simulink model "gm_sampleModel1406_3_sub"  (R2023a)
settings: Solver=VariableStepAuto  StartTime=0.0  StopTime=10.0  RelTol=1e-3
libraries: hdlsllib x2
settings Model: Creator=user1  LastModifiedBy=user1
settings OptimizationCC: BlockReduction=off  ConditionallyExecuteInputs=off
settings DebuggingCC: InheritedTsInSrcMsg=none

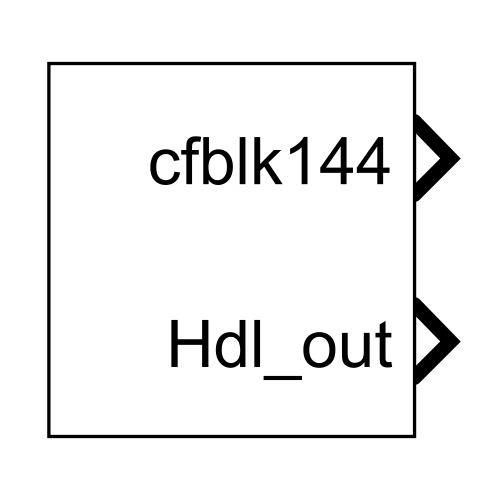
[thumbnail: Simulink's stored preview of the top-level diagram]
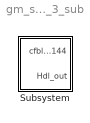
== system gm_sampleModel1406_3_sub ==
  Subsystem : Subsystem

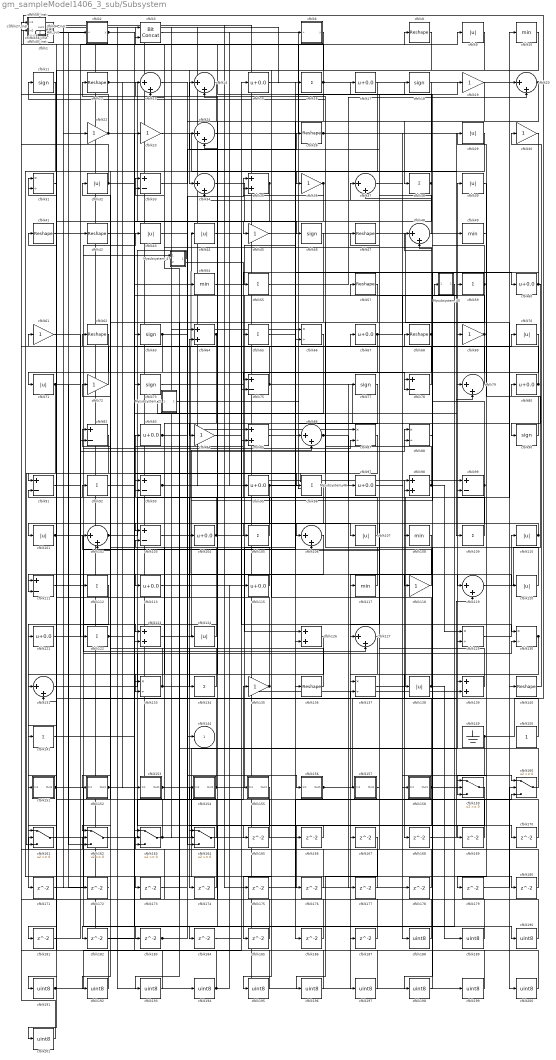
== system gm_sampleModel1406_3_sub/Subsystem ==
  Mysubsystem_21 : Subsystem
  Mysubsystem_40 : Subsystem
  Mysubsystem_46 : Subsystem
  Mysubsystem_47 : Subsystem
  cfblk1 : hdlsllib/Logic and Bit Operations/Interval Test  IntervalClosedRight=on  uplimit=0.5  IntervalClosedLeft=on  lowlimit=-0.5  OutDataTypeStr=uint8
  cfblk{10,49,54,108,117} (5 alike) : MinMax  OutDataTypeStr=uint8
  cfblk{9,29,32,39,43..44,70..71,101,107,110,120,124,138} (14 alike) : Abs  OutDataTypeStr=uint8  SaturateOnIntegerOverflow=off
  cfblk{13..14,20,24,34,37,48,79,86,102,106,119,127,131} (14 alike) : Sum  Inputs=|++  OutDataTypeStr=uint8
  cfblk{33,75,78,82,91,93,99,103,111} (9 alike) : Sum  Inputs=+-  OutDataTypeStr=uint8
  cfblk{15,17,60,67,80,83,95,97,104,113,115,121} (12 alike) : Bias  Bias=0.0  SaturateOnIntegerOverflow=off
  cfblk{16,38,55,59,65,92,96,105,109,112,122,134,141} (13 alike) : Sum  Inputs=+  OutDataTypeStr=uint8
  cfblk{11,18,46,63,73,77,90} (7 alike) : Signum
  cfblk114_inst : Subsystem
  cfblk116_inst : Subsystem
  cfblk{19,22..23,30,36,45,61,69,72,84,118,135} (12 alike) : Gain  OutDataTypeStr=uint8
  cfblk{8,12,26,41..42,47,57,62,68,136,140} (11 alike) : Reshape
  cfblk{35,64,85,98,123,126,139} (7 alike) : Sum  OutDataTypeStr=uint8
  cfblk128_inst : Subsystem
  cfblk{31,66,87..88,129..130,133,137} (8 alike) : Product  Inputs=*/  OutDataTypeStr=uint8  RndMeth=Zero  SaturateOnIntegerOverflow=on
  cfblk132_inst : Subsystem
  cfblk149 : Ground
  cfblk150 : Constant  OutDataTypeStr=uint8  SampleTime=-1
  cfblk151 : Subsystem
  cfblk152 : Subsystem
  cfblk153 : Subsystem
  cfblk154 : Subsystem
  cfblk155 : Subsystem
  cfblk156 : Subsystem
  cfblk157 : Subsystem
  cfblk158 : Subsystem
  cfblk{159..164} (6 alike) : Switch  OutDataTypeStr=uint8  SaturateOnIntegerOverflow=off  InputSameDT=off
  cfblk{165..187} (23 alike) : Delay  SampleTime=1
  cfblk{188..201} (14 alike) : DataTypeConversion  OutDataTypeStr=uint8  SaturateOnIntegerOverflow=off  RndMeth=Floor
  cfblk2 : Subsystem  mask(Compare To Constant){relop=<=, const=double(3), OutDataTypeStr=uint8, ZeroCross=on}
      mask prompts: relop "Simulink:masks:Operator_MP"; const "Simulink:masks:ConstantValue_MP"; OutDataTypeStr "Simulink:masks:OutputDataType_MP"; ZeroCross "Simulink:masks:EnableZerocrossingDetection_MP"
      mask help: Simulink:masks:CompareToConstant_MD
      mask init:
      | OutDataTypeStr = 'uint8';
      | ZeroCross = 'on';
      | blkName = 'sampleModel1406_3_sub/Subsystem/cfblk2';
      | const = double(3);
      | const_str = '3.0';
      | const_val = double(3);
      | relop = '<=';
      | setValue = 'fixdt(0, 8)';
      | str = '<= 3';
      mask TypeOptions relop: == | ~= | < | <= | >= | >
      mask TypeOptions OutDataTypeStr: Simulink:masks:uint8 | Simulink:masks:boolean
      mask Callback ZeroCross: sl('zeroCrossEnable', gcbh);
      mask Display: disp(str)
  cfblk25_inst : Subsystem
  cfblk27_inst : Subsystem
  cfblk3 : hdlsllib/Logic and Bit Operations/Bit Concat  numInputs=2
  cfblk4 : Constant  Value=0  OutDataTypeStr=uint8  SampleTime=1
  cfblk40_inst : Subsystem
  cfblk5 : Constant  Value=0  OutDataTypeStr=uint8  SampleTime=1
  cfblk56_inst : Subsystem
  cfblk58_inst : Subsystem
  cfblk6 : Subsystem  mask(Compare To Zero){relop=<=, OutDataTypeStr=uint8, ZeroCross=on}
      mask prompts: relop "Simulink:masks:Operator_MP"; OutDataTypeStr "Simulink:masks:OutputDataType_MP"; ZeroCross "Simulink:masks:EnableZerocrossingDetection_MP"
      mask help: Simulink:masks:CompareToZero_MD
      mask init:
      | OutDataTypeStr = 'uint8';
      | ZeroCross = 'on';
      | blkName = 'sampleModel1406_3_sub/Subsystem/cfblk6';
      | relop = '<=';
      | setValue = 'fixdt(0, 8)';
      mask TypeOptions relop: == | ~= | < | <= | >= | >
      mask TypeOptions OutDataTypeStr: Simulink:masks:uint8 | Simulink:masks:boolean
      mask Callback ZeroCross: sl('zeroCrossEnable', gcbh);
      mask Display: disp([relop,' 0'])
  cfblk94_inst : Subsystem
  cfblk144 : Outport  OutDataTypeStr=uint8  SampleTime=1  VectorParamsAs1DForOutWhenUnconnected=off
  Hdl_out : Outport  Port=2  OutDataTypeStr=uint8  SampleTime=1
  wires:
  Mysubsystem_21/1(Out1) -> Mysubsystem_46/2(In2)
  Mysubsystem_40/1(Out1) -> cfblk182/1
  Mysubsystem_46/1(Out1) -> Mysubsystem_47/2(In2)
  Mysubsystem_47/1(Out1) -> cfblk165/1
  cfblk1/1 -> cfblk2/1(u)
  cfblk10/1 -> cfblk34/1
  cfblk101/1 -> cfblk43/1, cfblk127/2, cfblk123/1, Mysubsystem_47/1(In1)
  cfblk102/1 -> cfblk98/1, cfblk174/1
  cfblk103/1 -> cfblk37/2
  cfblk104/1 -> cfblk91/2, cfblk57/1, cfblk126/1
  cfblk105/1 -> cfblk83/1
  cfblk106/1 -> cfblk111/2
  cfblk107/1 -> cfblk65/1
  cfblk108/1 -> cfblk197/1
  cfblk109/1 -> cfblk39/1
  cfblk11/1 -> cfblk173/1
  cfblk110/1 -> cfblk106/1, cfblk105/1
  cfblk111/1 -> cfblk87/2
  cfblk112/1 -> cfblk171/1
  cfblk113/1 -> cfblk19/1
  cfblk114_inst/1(out1) -> cfblk199/1
  cfblk115/1 -> cfblk14/1
  cfblk116_inst/1(out1) -> cfblk20/1
  cfblk117/1 -> cfblk12/1
  cfblk118/1 -> cfblk102/1
  cfblk119/1 -> cfblk80/1
  cfblk12/1 -> cfblk186/1, cfblk153/1(In1)
  cfblk120/1 -> cfblk13/1
  cfblk121/1 -> cfblk86/1
  cfblk122/1 -> cfblk93/2, cfblk85/1
  cfblk123/1 -> cfblk86/2
  cfblk124/1 -> cfblk62/1
  cfblk126/1 -> cfblk131/2
  cfblk127/1 -> cfblk187/1
  cfblk128_inst/1(out1) -> cfblk97/1
  cfblk129/1 -> cfblk110/1
  cfblk13/1 -> cfblk144/1
  cfblk130/1 -> cfblk168/1, cfblk167/1, cfblk137/1
  cfblk131/1 -> cfblk130/2
  cfblk132_inst/1(out1) -> cfblk87/1
  cfblk133/1 -> cfblk44/1, cfblk92/1
  cfblk134/1 -> cfblk93/1
  cfblk135/1 -> cfblk64/2, cfblk61/1
  cfblk136/1 -> cfblk72/1
  cfblk137/1 -> cfblk10/1
  cfblk138/1 -> cfblk95/1, cfblk189/1
  cfblk139/1 -> cfblk106/2
  cfblk14/1 -> cfblk113/1
  cfblk140/1 -> cfblk30/1
  cfblk141/1 -> cfblk63/1
  cfblk149/1 -> cfblk94_inst/1(in1), cfblk159/3
  cfblk15/1 -> cfblk200/1
  cfblk150/1 -> cfblk128_inst/1(in1)
  cfblk151/1(Out1) -> cfblk183/1, cfblk137/2
  cfblk152/1(Out1) -> cfblk68/1, cfblk190/1
  cfblk153/1(Out1) -> cfblk69/1, cfblk185/1
  cfblk154/1(Out1) -> cfblk82/1, cfblk66/2
  cfblk155/1(Out1) -> cfblk184/1
  cfblk156/1(Out1) -> cfblk139/1, cfblk157/1(In1)
  cfblk157/1(Out1) -> cfblk47/1
  cfblk158/1(Out1) -> cfblk98/2, cfblk195/1, cfblk159/2
  cfblk159/1 -> cfblk176/1
  cfblk16/1 -> cfblk116_inst/2(in2), cfblk104/1
  cfblk160/1 -> cfblk33/1
  cfblk161/1 -> cfblk88/1
  cfblk162/1 -> cfblk135/1
  cfblk163/1 -> cfblk75/2, cfblk41/1
  cfblk164/1 -> cfblk32/1
  cfblk165/1 -> cfblk33/2
  cfblk166/1 -> cfblk164/1
  cfblk167/1 -> cfblk196/1
  cfblk168/1 -> cfblk119/2
  cfblk169/1 -> cfblk103/2
  cfblk17/1 -> cfblk121/1
  cfblk170/1 -> cfblk24/2
  cfblk171/1 -> cfblk129/2
  cfblk172/1 -> cfblk1/1
  cfblk173/1 -> cfblk99/2
  cfblk174/1 -> cfblk58_inst/2(in2)
  cfblk175/1 -> cfblk160/3
  cfblk176/1 -> cfblk162/2
  cfblk177/1 -> cfblk14/2
  cfblk178/1 -> cfblk37/1
  cfblk179/1 -> cfblk160/2
  cfblk18/1 -> cfblk152/1(In1)
  cfblk180/1 -> cfblk161/2
  cfblk181/1 -> cfblk88/2
  cfblk182/1 -> cfblk79/1
  cfblk183/1 -> cfblk35/1, Hdl_out/1
  cfblk184/1 -> cfblk85/2
  cfblk185/1 -> cfblk163/2
  cfblk186/1 -> cfblk163/1
  cfblk187/1 -> cfblk116_inst/1(in1)
  cfblk188/1 -> cfblk154/1(In1)
  cfblk189/1 -> cfblk3/1
  cfblk19/1 -> cfblk38/1
  cfblk190/1 -> cfblk3/2
  cfblk191/1 -> cfblk15/1, cfblk23/1
  cfblk192/1 -> cfblk31/1
  cfblk193/1 -> cfblk31/2
  cfblk194/1 -> cfblk56_inst/1(in1), cfblk115/1
  cfblk195/1 -> cfblk40_inst/1(in1)
  cfblk196/1 -> cfblk40_inst/2(in2)
  cfblk197/1 -> cfblk27_inst/1(in1)
  cfblk198/1 -> cfblk108/1
  cfblk199/1 -> cfblk27_inst/2(in2)
  cfblk2/1(y) -> cfblk46/1, cfblk45/1
  cfblk20/1 -> cfblk126/2, cfblk84/1
  cfblk200/1 -> cfblk114_inst/1(in1)
  cfblk201/1 -> cfblk114_inst/2(in2)
  cfblk22/1 -> cfblk94_inst/2(in2), cfblk132_inst/2(in2), cfblk180/1, cfblk96/1
  cfblk23/1 -> cfblk109/1
  cfblk24/1 -> cfblk9/1
  cfblk25_inst/1(out1) -> cfblk166/1
  cfblk26/1 -> cfblk79/2, cfblk158/1(In1)
  cfblk27_inst/1(out1) -> cfblk56_inst/2(in2), cfblk66/1
  cfblk29/1 -> cfblk36/1
  cfblk3/1 -> cfblk188/1
  cfblk30/1 -> cfblk198/1
  cfblk31/1 -> cfblk191/1
  cfblk32/1 -> cfblk73/1, cfblk132_inst/1(in1)
  cfblk33/1 -> cfblk26/1
  cfblk34/1 -> cfblk136/1
  cfblk35/1 -> cfblk192/1, cfblk162/1
  cfblk36/1 -> cfblk71/1, cfblk35/2
  cfblk37/1 -> cfblk160/1
  cfblk38/1 -> cfblk161/1, cfblk128_inst/2(in2)
  cfblk39/1 -> cfblk159/1
  cfblk4/1 -> cfblk139/2, cfblk155/1(In1)
  cfblk40_inst/1(out1) -> cfblk194/1
  cfblk41/1 -> cfblk42/1
  cfblk42/1 -> cfblk54/1
  cfblk43/1 -> cfblk117/1
  cfblk44/1 -> cfblk107/1
  cfblk45/1 -> cfblk60/1
  cfblk46/1 -> cfblk133/2
  cfblk47/1 -> cfblk140/1
  cfblk48/1 -> cfblk24/1
  cfblk49/1 -> cfblk179/1
  cfblk5/1 -> cfblk22/1, cfblk178/1
  cfblk54/1 -> cfblk16/1
  cfblk55/1 -> cfblk20/2
  cfblk56_inst/1(out1) -> cfblk172/1, cfblk112/1
  cfblk57/1 -> cfblk103/1
  cfblk58_inst/1(out1) -> cfblk99/1
  cfblk59/1 -> cfblk34/2, cfblk102/2, cfblk175/1, Mysubsystem_46/1(In1)
  cfblk6/1(y) -> cfblk151/1(In1)
  cfblk60/1 -> cfblk90/1, cfblk55/1
  cfblk61/1 -> cfblk122/1
  cfblk62/1 -> cfblk111/1
  cfblk63/1 -> cfblk131/1, cfblk169/1
  cfblk64/1 -> cfblk133/1, cfblk134/1
  cfblk65/1 -> cfblk78/2
  cfblk66/1 -> Mysubsystem_21/1(In1)
  cfblk67/1 -> cfblk193/1, cfblk59/1
  cfblk68/1 -> cfblk163/3, cfblk13/2
  cfblk69/1 -> cfblk17/1, cfblk164/3
  cfblk70/1 -> cfblk101/1
  cfblk71/1 -> cfblk82/2, cfblk162/3, cfblk161/3
  cfblk72/1 -> cfblk25_inst/1(in1)
  cfblk73/1 -> cfblk78/1
  cfblk75/1 -> cfblk25_inst/2(in2), cfblk138/1
  cfblk77/1 -> cfblk124/1
  cfblk78/1 -> cfblk67/1
  cfblk79/1 -> cfblk64/1
  cfblk8/1 -> cfblk75/1
  cfblk80/1 -> cfblk58_inst/1(in1), cfblk48/2
  cfblk82/1 -> cfblk201/1
  cfblk83/1 -> cfblk170/1, cfblk156/1(In1)
  cfblk84/1 -> cfblk70/1
  cfblk85/1 -> cfblk119/1
  cfblk86/1 -> cfblk177/1, cfblk118/1
  cfblk87/1 -> cfblk141/1
  cfblk88/1 -> cfblk48/1
  cfblk9/1 -> cfblk91/1
  cfblk90/1 -> cfblk29/1
  cfblk91/1 -> cfblk8/1
  cfblk92/1 -> Mysubsystem_40/1(In1)
  cfblk93/1 -> cfblk130/1, cfblk6/1(u)
  cfblk94_inst/1(out1) -> cfblk49/1
  cfblk95/1 -> cfblk164/2, cfblk123/2
  cfblk96/1 -> cfblk77/1, cfblk181/1
  cfblk97/1 -> cfblk120/1
  cfblk98/1 -> cfblk11/1, cfblk129/1
  cfblk99/1 -> cfblk18/1, cfblk127/1

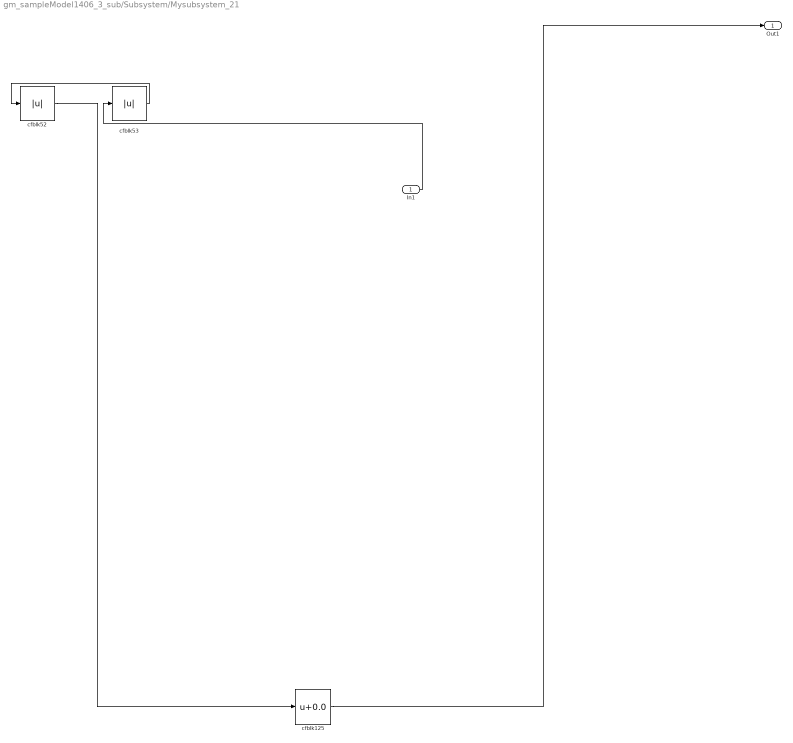
== system gm_sampleModel1406_3_sub/Subsystem/Mysubsystem_21 ==
  In1 : Inport  OutDataTypeStr=uint8  PortDimensions=1  SampleTime=1
  cfblk125 : Bias  Bias=0.0  SaturateOnIntegerOverflow=off
  cfblk52 : Abs  SaturateOnIntegerOverflow=off
  cfblk53 : Abs  SaturateOnIntegerOverflow=off
  Out1 : Outport  SampleTime=1
  wires:
  In1/1 -> cfblk53/1
  cfblk125/1 -> Out1/1
  cfblk52/1 -> cfblk125/1
  cfblk53/1 -> cfblk52/1

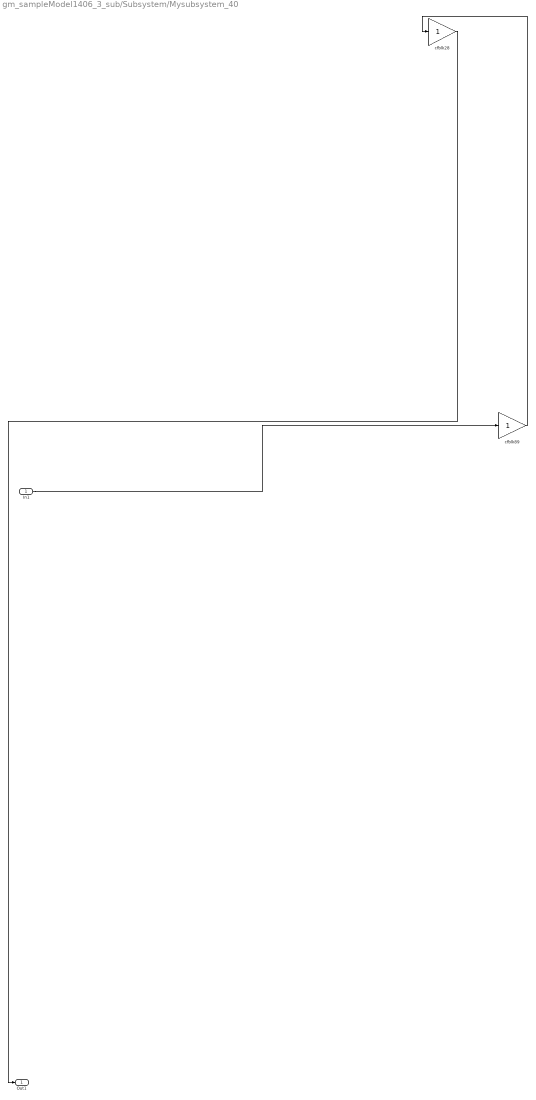
== system gm_sampleModel1406_3_sub/Subsystem/Mysubsystem_40 ==
  In1 : Inport  OutDataTypeStr=uint8  PortDimensions=1  SampleTime=1
  cfblk28 : Gain
  cfblk89 : Gain
  Out1 : Outport  SampleTime=1
  wires:
  In1/1 -> cfblk89/1
  cfblk28/1 -> Out1/1
  cfblk89/1 -> cfblk28/1

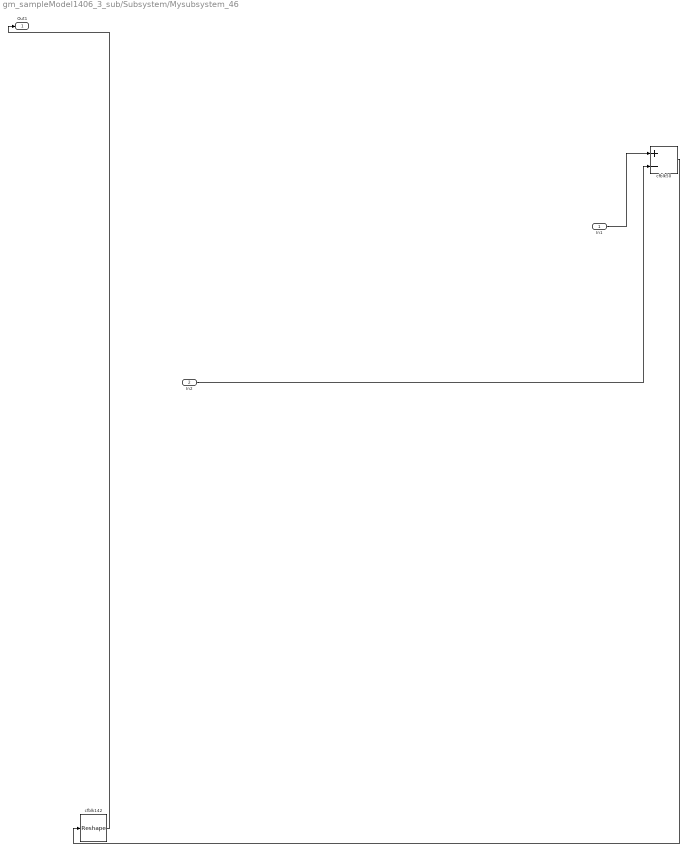
== system gm_sampleModel1406_3_sub/Subsystem/Mysubsystem_46 ==
  In1 : Inport  OutDataTypeStr=uint8  PortDimensions=1  SampleTime=1
  In2 : Inport  Port=2  OutDataTypeStr=uint8  PortDimensions=1  SampleTime=1
  cfblk142 : Reshape
  cfblk50 : Sum  Inputs=+-
  Out1 : Outport  SampleTime=1
  wires:
  In1/1 -> cfblk50/1
  In2/1 -> cfblk50/2
  cfblk142/1 -> Out1/1
  cfblk50/1 -> cfblk142/1

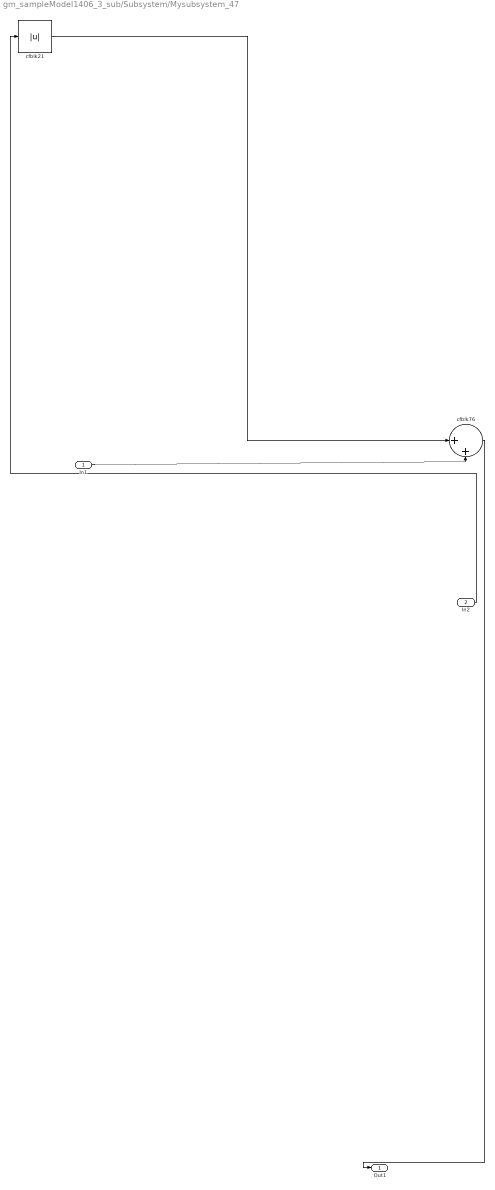
== system gm_sampleModel1406_3_sub/Subsystem/Mysubsystem_47 ==
  In1 : Inport  OutDataTypeStr=uint8  PortDimensions=1  SampleTime=1
  In2 : Inport  Port=2  OutDataTypeStr=uint8  PortDimensions=1  SampleTime=1
  cfblk21 : Abs  SaturateOnIntegerOverflow=off
  cfblk76 : Sum  Inputs=|++
  Out1 : Outport  SampleTime=1
  wires:
  In1/1 -> cfblk76/2
  In2/1 -> cfblk21/1
  cfblk21/1 -> cfblk76/1
  cfblk76/1 -> Out1/1

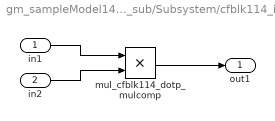
== system gm_sampleModel1406_3_sub/Subsystem/cfblk114_inst ==
  in1 : Inport  OutDataTypeStr=uint8  SampleTime=1
  in2 : Inport  Port=2  OutDataTypeStr=uint8  SampleTime=1
  mul_cfblk114_dotp_mulcomp : Product  Inputs=**  OutDataTypeStr=uint8  SampleTime=1
  out1 : Outport  OutDataTypeStr=uint8  SampleTime=1
  wires:
  in1/1 -> mul_cfblk114_dotp_mulcomp/1
  in2/1 -> mul_cfblk114_dotp_mulcomp/2
  mul_cfblk114_dotp_mulcomp/1 -> out1/1

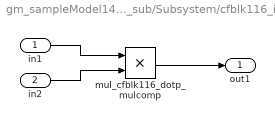
== system gm_sampleModel1406_3_sub/Subsystem/cfblk116_inst ==
  in1 : Inport  OutDataTypeStr=uint8  SampleTime=1
  in2 : Inport  Port=2  OutDataTypeStr=uint8  SampleTime=1
  mul_cfblk116_dotp_mulcomp : Product  Inputs=**  OutDataTypeStr=uint8  SampleTime=1
  out1 : Outport  OutDataTypeStr=uint8  SampleTime=1
  wires:
  in1/1 -> mul_cfblk116_dotp_mulcomp/1
  in2/1 -> mul_cfblk116_dotp_mulcomp/2
  mul_cfblk116_dotp_mulcomp/1 -> out1/1

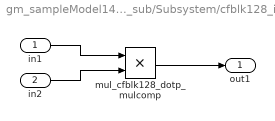
== system gm_sampleModel1406_3_sub/Subsystem/cfblk128_inst ==
  in1 : Inport  OutDataTypeStr=uint8  SampleTime=1
  in2 : Inport  Port=2  OutDataTypeStr=uint8  SampleTime=1
  mul_cfblk128_dotp_mulcomp : Product  Inputs=**  OutDataTypeStr=uint8  SampleTime=1
  out1 : Outport  OutDataTypeStr=uint8  SampleTime=1
  wires:
  in1/1 -> mul_cfblk128_dotp_mulcomp/1
  in2/1 -> mul_cfblk128_dotp_mulcomp/2
  mul_cfblk128_dotp_mulcomp/1 -> out1/1

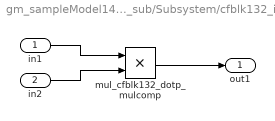
== system gm_sampleModel1406_3_sub/Subsystem/cfblk132_inst ==
  in1 : Inport  OutDataTypeStr=uint8  SampleTime=1
  in2 : Inport  Port=2  OutDataTypeStr=uint8  SampleTime=1
  mul_cfblk132_dotp_mulcomp : Product  Inputs=**  OutDataTypeStr=uint8  SampleTime=1
  out1 : Outport  OutDataTypeStr=uint8  SampleTime=1
  wires:
  in1/1 -> mul_cfblk132_dotp_mulcomp/1
  in2/1 -> mul_cfblk132_dotp_mulcomp/2
  mul_cfblk132_dotp_mulcomp/1 -> out1/1

== system gm_sampleModel1406_3_sub/Subsystem/cfblk151 ==
  In1 : Inport  OutDataTypeStr=uint8  PortDimensions=1  SampleTime=1
  Out1 : Outport  SampleTime=1
  wires:
  In1/1 -> Out1/1

== system gm_sampleModel1406_3_sub/Subsystem/cfblk152 ==
  In1 : Inport  OutDataTypeStr=uint8  PortDimensions=1  SampleTime=1
  Out1 : Outport  SampleTime=1
  wires:
  In1/1 -> Out1/1

== system gm_sampleModel1406_3_sub/Subsystem/cfblk153 ==
  In1 : Inport  OutDataTypeStr=uint8  PortDimensions=1  SampleTime=1
  Out1 : Outport  SampleTime=1
  wires:
  In1/1 -> Out1/1

== system gm_sampleModel1406_3_sub/Subsystem/cfblk154 ==
  In1 : Inport  OutDataTypeStr=uint8  PortDimensions=1  SampleTime=1
  Out1 : Outport  SampleTime=1
  wires:
  In1/1 -> Out1/1

== system gm_sampleModel1406_3_sub/Subsystem/cfblk155 ==
  In1 : Inport  OutDataTypeStr=uint8  PortDimensions=1  SampleTime=1
  Out1 : Outport  SampleTime=1
  wires:
  In1/1 -> Out1/1

== system gm_sampleModel1406_3_sub/Subsystem/cfblk156 ==
  In1 : Inport  OutDataTypeStr=uint8  PortDimensions=1  SampleTime=1
  Out1 : Outport  SampleTime=1
  wires:
  In1/1 -> Out1/1

== system gm_sampleModel1406_3_sub/Subsystem/cfblk157 ==
  In1 : Inport  OutDataTypeStr=uint8  PortDimensions=1  SampleTime=1
  Out1 : Outport  SampleTime=1
  wires:
  In1/1 -> Out1/1

== system gm_sampleModel1406_3_sub/Subsystem/cfblk158 ==
  In1 : Inport  OutDataTypeStr=uint8  PortDimensions=1  SampleTime=1
  Out1 : Outport  SampleTime=1
  wires:
  In1/1 -> Out1/1

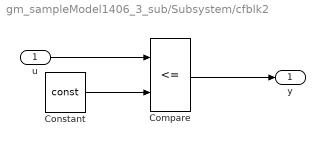
== system gm_sampleModel1406_3_sub/Subsystem/cfblk2 ==
  u : Inport  OutDataTypeStr=uint8  SampleTime=1
  Compare : RelationalOperator  Operator=<=  OutDataTypeStr=fixdt(0, 8)
  Constant : Constant  DisableCoverage=on  Value=const  OutDataTypeStr=Inherit: Inherit via back propagation  SampleTime=-1
  y : Outport  SampleTime=1
  wires:
  u/1 -> Compare/1
  Compare/1 -> y/1
  Constant/1 -> Compare/2

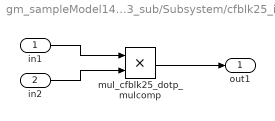
== system gm_sampleModel1406_3_sub/Subsystem/cfblk25_inst ==
  in1 : Inport  OutDataTypeStr=uint8  SampleTime=1
  in2 : Inport  Port=2  OutDataTypeStr=uint8  SampleTime=1
  mul_cfblk25_dotp_mulcomp : Product  Inputs=**  OutDataTypeStr=uint8  SampleTime=1
  out1 : Outport  OutDataTypeStr=uint8  SampleTime=1
  wires:
  in1/1 -> mul_cfblk25_dotp_mulcomp/1
  in2/1 -> mul_cfblk25_dotp_mulcomp/2
  mul_cfblk25_dotp_mulcomp/1 -> out1/1

== system gm_sampleModel1406_3_sub/Subsystem/cfblk27_inst ==
  in1 : Inport  OutDataTypeStr=uint8  SampleTime=1
  in2 : Inport  Port=2  OutDataTypeStr=uint8  SampleTime=1
  mul_cfblk27_dotp_mulcomp : Product  Inputs=**  OutDataTypeStr=uint8  SampleTime=1
  out1 : Outport  OutDataTypeStr=uint8  SampleTime=1
  wires:
  in1/1 -> mul_cfblk27_dotp_mulcomp/1
  in2/1 -> mul_cfblk27_dotp_mulcomp/2
  mul_cfblk27_dotp_mulcomp/1 -> out1/1

== system gm_sampleModel1406_3_sub/Subsystem/cfblk40_inst ==
  in1 : Inport  OutDataTypeStr=uint8  SampleTime=1
  in2 : Inport  Port=2  OutDataTypeStr=uint8  SampleTime=1
  mul_cfblk40_dotp_mulcomp : Product  Inputs=**  OutDataTypeStr=uint8  SampleTime=1
  out1 : Outport  OutDataTypeStr=uint8  SampleTime=1
  wires:
  in1/1 -> mul_cfblk40_dotp_mulcomp/1
  in2/1 -> mul_cfblk40_dotp_mulcomp/2
  mul_cfblk40_dotp_mulcomp/1 -> out1/1

== system gm_sampleModel1406_3_sub/Subsystem/cfblk56_inst ==
  in1 : Inport  OutDataTypeStr=uint8  SampleTime=1
  in2 : Inport  Port=2  OutDataTypeStr=uint8  SampleTime=1
  mul_cfblk56_dotp_mulcomp : Product  Inputs=**  OutDataTypeStr=uint8  SampleTime=1
  out1 : Outport  OutDataTypeStr=uint8  SampleTime=1
  wires:
  in1/1 -> mul_cfblk56_dotp_mulcomp/1
  in2/1 -> mul_cfblk56_dotp_mulcomp/2
  mul_cfblk56_dotp_mulcomp/1 -> out1/1

== system gm_sampleModel1406_3_sub/Subsystem/cfblk58_inst ==
  in1 : Inport  OutDataTypeStr=uint8  SampleTime=1
  in2 : Inport  Port=2  OutDataTypeStr=uint8  SampleTime=1
  mul_cfblk58_dotp_mulcomp : Product  Inputs=**  OutDataTypeStr=uint8  SampleTime=1
  out1 : Outport  OutDataTypeStr=uint8  SampleTime=1
  wires:
  in1/1 -> mul_cfblk58_dotp_mulcomp/1
  in2/1 -> mul_cfblk58_dotp_mulcomp/2
  mul_cfblk58_dotp_mulcomp/1 -> out1/1

== system gm_sampleModel1406_3_sub/Subsystem/cfblk6 ==
  u : Inport  OutDataTypeStr=uint8  SampleTime=1
  Compare : RelationalOperator  Operator=<=  OutDataTypeStr=fixdt(0, 8)
  Constant : Constant  DisableCoverage=on  Value=0  OutDataTypeStr=Inherit: Inherit via back propagation  SampleTime=-1  PreserveConstantTs=on
  y : Outport  SampleTime=1
  wires:
  u/1 -> Compare/1
  Compare/1 -> y/1
  Constant/1 -> Compare/2

== system gm_sampleModel1406_3_sub/Subsystem/cfblk94_inst ==
  in1 : Inport  OutDataTypeStr=uint8  SampleTime=1
  in2 : Inport  Port=2  OutDataTypeStr=uint8  SampleTime=1
  mul_cfblk94_dotp_mulcomp : Product  Inputs=**  OutDataTypeStr=uint8  SampleTime=1
  out1 : Outport  OutDataTypeStr=uint8  SampleTime=1
  wires:
  in1/1 -> mul_cfblk94_dotp_mulcomp/1
  in2/1 -> mul_cfblk94_dotp_mulcomp/2
  mul_cfblk94_dotp_mulcomp/1 -> out1/1
